simulink model "distributeSystemSim"  (R2017a)
settings: Solver=VariableStepAuto  StartTime=0.0  StopTime=200  RelTol=1e-3
libraries: simulink x3
settings Model: Creator=17423  LastModifiedBy=17423

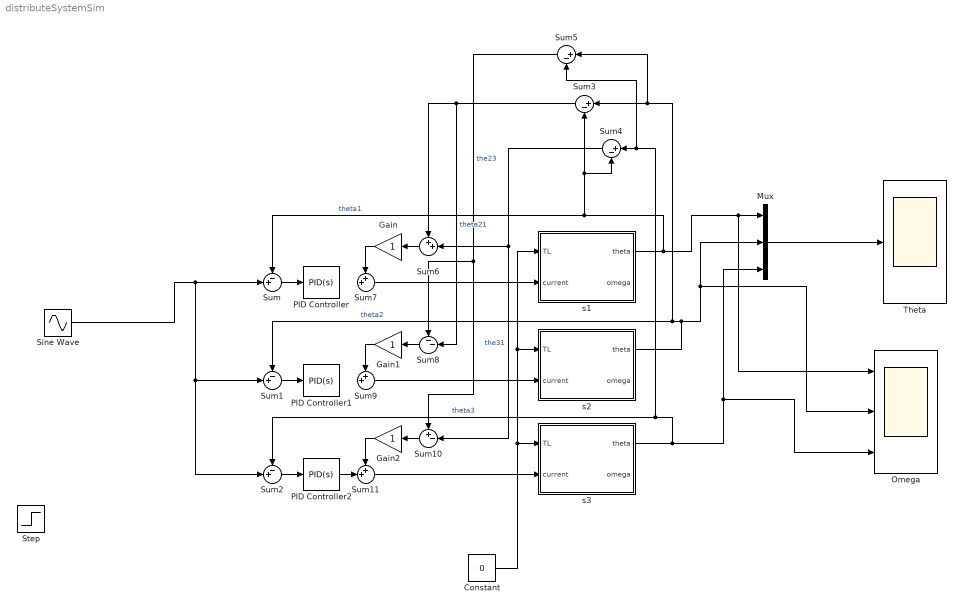
== system distributeSystemSim ==
  Constant : Constant  Value=0
  Gain : Gain
  Gain1 : Gain
  Gain2 : Gain
  Mux : Mux  Inputs=3
  Omega : Scope  NumInputPorts=3
  PID Controller : simulink/Continuous/PID Controller  Controller=PID  TimeDomain=Continuous-time  SampleTime=-1  IntegratorMethod=Forward Euler  FilterMethod=Forward Euler  Form=Parallel  UseFilter=on  ControllerParametersSource=internal  P=0.1  I=0  D=16  N=100  InitialConditionSource=internal  InitialConditionForIntegrator=0  InitialConditionForFilter=0  ExternalReset=none  LimitOutput=off  UpperSaturationLimit=inf  LowerSaturationLimit=-inf  LinearizeAsGain=on  AntiWindupMode=none  Kb=1  TrackingMode=off  Kt=1  PParamMin=[]  PParamMax=[]  IParamMin=[]  IParamMax=[]  DParamMin=[]  DParamMax=[]  NParamMin=[]  NParamMax=[]  KbParamMin=[]  KbParamMax=[]  KtParamMin=[]  KtParamMax=[]  POutMin=[]  POutMax=[]  IOutMin=[]  IOutMax=[]  DOutMin=[]  DOutMax=[]  NOutMin=[]  NOutMax=[]  KbOutMin=[]  KbOutMax=[]  KtOutMin=[]  KtOutMax=[]  IntegratorOutMin=[]  IntegratorOutMax=[]  FilterOutMin=[]  FilterOutMax=[]  SumOutMin=[]  SumOutMax=[]  SumI1OutMin=[]  SumI1OutMax=[]  SumI2OutMin=[]  SumI2OutMax=[]  SumI3OutMin=[]  SumI3OutMax=[]  SumDOutMin=[]  SumDOutMax=[]  SaturationOutMin=[]  SaturationOutMax=[]  IntegratorContinuousStateAttributes=''  IntegratorStateMustResolveToSignalObject=off  IntegratorRTWStateStorageClass=Auto  FilterContinuousStateAttributes=''  FilterStateMustResolveToSignalObject=off  FilterRTWStateStorageClass=Auto  DifferentiatorICPrevScaledInput=0  DifferentiatorOutMin=[]  DifferentiatorOutMax=[]  InitialConditionSetting=State (most efficient)
  PID Controller1 : simulink/Continuous/PID Controller  Controller=PID  TimeDomain=Continuous-time  SampleTime=-1  IntegratorMethod=Forward Euler  FilterMethod=Forward Euler  Form=Parallel  UseFilter=on  ControllerParametersSource=internal  P=0.1  I=0  D=16  N=100  InitialConditionSource=internal  InitialConditionForIntegrator=0  InitialConditionForFilter=0  ExternalReset=none  LimitOutput=off  UpperSaturationLimit=inf  LowerSaturationLimit=-inf  LinearizeAsGain=on  AntiWindupMode=none  Kb=1  TrackingMode=off  Kt=1  PParamMin=[]  PParamMax=[]  IParamMin=[]  IParamMax=[]  DParamMin=[]  DParamMax=[]  NParamMin=[]  NParamMax=[]  KbParamMin=[]  KbParamMax=[]  KtParamMin=[]  KtParamMax=[]  POutMin=[]  POutMax=[]  IOutMin=[]  IOutMax=[]  DOutMin=[]  DOutMax=[]  NOutMin=[]  NOutMax=[]  KbOutMin=[]  KbOutMax=[]  KtOutMin=[]  KtOutMax=[]  IntegratorOutMin=[]  IntegratorOutMax=[]  FilterOutMin=[]  FilterOutMax=[]  SumOutMin=[]  SumOutMax=[]  SumI1OutMin=[]  SumI1OutMax=[]  SumI2OutMin=[]  SumI2OutMax=[]  SumI3OutMin=[]  SumI3OutMax=[]  SumDOutMin=[]  SumDOutMax=[]  SaturationOutMin=[]  SaturationOutMax=[]  IntegratorContinuousStateAttributes=''  IntegratorStateMustResolveToSignalObject=off  IntegratorRTWStateStorageClass=Auto  FilterContinuousStateAttributes=''  FilterStateMustResolveToSignalObject=off  FilterRTWStateStorageClass=Auto  DifferentiatorICPrevScaledInput=0  DifferentiatorOutMin=[]  DifferentiatorOutMax=[]  InitialConditionSetting=State (most efficient)
  PID Controller2 : simulink/Continuous/PID Controller  Controller=PID  TimeDomain=Continuous-time  SampleTime=-1  IntegratorMethod=Forward Euler  FilterMethod=Forward Euler  Form=Parallel  UseFilter=on  ControllerParametersSource=internal  P=0.1  I=0  D=16  N=100  InitialConditionSource=internal  InitialConditionForIntegrator=0  InitialConditionForFilter=0  ExternalReset=none  LimitOutput=off  UpperSaturationLimit=inf  LowerSaturationLimit=-inf  LinearizeAsGain=on  AntiWindupMode=none  Kb=1  TrackingMode=off  Kt=1  PParamMin=[]  PParamMax=[]  IParamMin=[]  IParamMax=[]  DParamMin=[]  DParamMax=[]  NParamMin=[]  NParamMax=[]  KbParamMin=[]  KbParamMax=[]  KtParamMin=[]  KtParamMax=[]  POutMin=[]  POutMax=[]  IOutMin=[]  IOutMax=[]  DOutMin=[]  DOutMax=[]  NOutMin=[]  NOutMax=[]  KbOutMin=[]  KbOutMax=[]  KtOutMin=[]  KtOutMax=[]  IntegratorOutMin=[]  IntegratorOutMax=[]  FilterOutMin=[]  FilterOutMax=[]  SumOutMin=[]  SumOutMax=[]  SumI1OutMin=[]  SumI1OutMax=[]  SumI2OutMin=[]  SumI2OutMax=[]  SumI3OutMin=[]  SumI3OutMax=[]  SumDOutMin=[]  SumDOutMax=[]  SaturationOutMin=[]  SaturationOutMax=[]  IntegratorContinuousStateAttributes=''  IntegratorStateMustResolveToSignalObject=off  IntegratorRTWStateStorageClass=Auto  FilterContinuousStateAttributes=''  FilterStateMustResolveToSignalObject=off  FilterRTWStateStorageClass=Auto  DifferentiatorICPrevScaledInput=0  DifferentiatorOutMin=[]  DifferentiatorOutMax=[]  InitialConditionSetting=State (most efficient)
  Sine Wave : Sin  Amplitude=2  Frequency=0.2  SampleTime=0
  Step : Step  Time=0  SampleTime=0
  Sum : Sum  Inputs=-+|
  Sum1 : Sum  Inputs=-+|
  Sum10 : Sum  Inputs=+-|
  Sum{6..7,9,11} (4 alike) : Sum  Inputs=++|
  Sum2 : Sum  Inputs=-+|
  Sum3 : Sum  Inputs=|+-
  Sum4 : Sum  Inputs=|+-
  Sum5 : Sum  Inputs=|+-
  Sum8 : Sum  Inputs=--|
  Theta : Scope
  s1 : Subsystem
  s2 : Subsystem
  s3 : Subsystem
  wires:
  Constant/1 -> s1/1(TL), s2/1(TL), s3/1(TL)
  Mux/1 -> Theta/1
  Sum/1 -> PID Controller/1
  s1/1(theta) -> Omega/1, Mux/1, Sum/1, Sum4/2, Sum3/2  "theta1"
  Sine Wave/1 -> Sum2/2, Sum1/2, Sum/2
  s2/1(theta) -> Omega/2, Mux/2, Sum5/1, Sum3/1, Sum1/1  "theta2"
  Sum1/1 -> PID Controller1/1
  s3/1(theta) -> Omega/3, Mux/3, Sum5/2, Sum4/1, Sum2/1  "theta3"
  Sum2/1 -> PID Controller2/1
  Sum3/1 -> Sum8/2, Sum6/1  "theta21"
  Sum4/1 -> Sum10/2, Sum6/2  "the31"
  Sum6/1 -> Gain/1
  Gain/1 -> Sum7/1
  Sum7/1 -> s1/2(current)
  PID Controller2/1 -> Sum11/2
  Gain2/1 -> Sum11/1
  Gain1/1 -> Sum9/1
  Sum5/1 -> Sum10/1, Sum8/1  "the23"
  Sum8/1 -> Gain1/1
  Sum9/1 -> s2/2(current)
  Sum10/1 -> Gain2/1
  Sum11/1 -> s3/2(current)

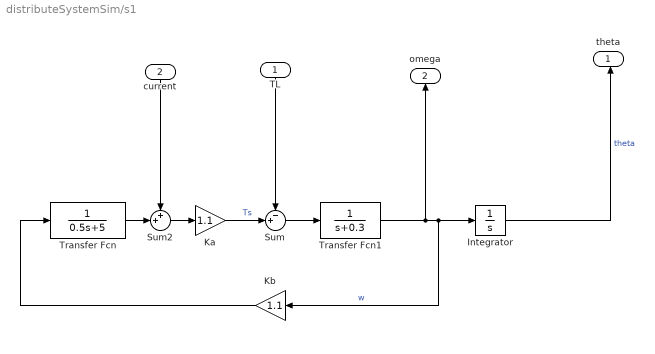
== system distributeSystemSim/s1 ==
  TL : Inport
  current : Inport  Port=2
  Integrator : Integrator  InitialCondition=-1
  Ka : Gain  Gain=1.1
  Kb : Gain  Gain=1.1
  Sum : Sum  Inputs=-+|
  Sum2 : Sum  Inputs=++|
  Transfer Fcn : TransferFcn  Denominator=[0.5 5]
  Transfer Fcn1 : TransferFcn  Denominator=[1 0.3]
  theta : Outport
  omega : Outport  Port=2
  wires:
  current/1 -> Sum2/1
  Sum2/1 -> Ka/1
  Ka/1 -> Sum/2  "Ts"
  Sum/1 -> Transfer Fcn1/1
  TL/1 -> Sum/1
  Transfer Fcn1/1 -> omega/1, Kb/1, Integrator/1  "w"
  Transfer Fcn/1 -> Sum2/2
  Kb/1 -> Transfer Fcn/1
  Integrator/1 -> theta/1  "theta"

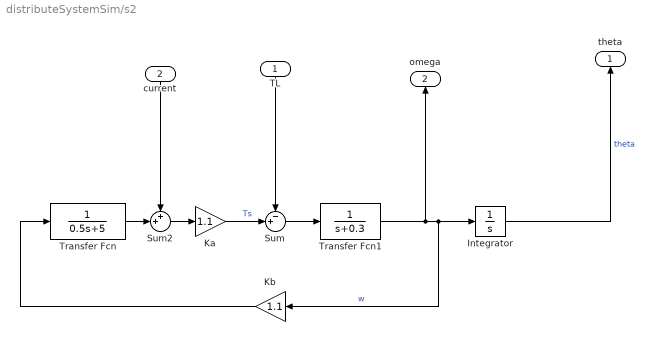
== system distributeSystemSim/s2 ==
  TL : Inport
  current : Inport  Port=2
  Integrator : Integrator  InitialCondition=-2
  Ka : Gain  Gain=1.1
  Kb : Gain  Gain=1.1
  Sum : Sum  Inputs=-+|
  Sum2 : Sum  Inputs=++|
  Transfer Fcn : TransferFcn  Denominator=[0.5 5]
  Transfer Fcn1 : TransferFcn  Denominator=[1 0.3]
  theta : Outport
  omega : Outport  Port=2
  wires:
  Integrator/1 -> theta/1  "theta"
  Kb/1 -> Transfer Fcn/1
  Transfer Fcn/1 -> Sum2/2
  Transfer Fcn1/1 -> Integrator/1, Kb/1, omega/1  "w"
  TL/1 -> Sum/1
  Sum/1 -> Transfer Fcn1/1
  Ka/1 -> Sum/2  "Ts"
  Sum2/1 -> Ka/1
  current/1 -> Sum2/1

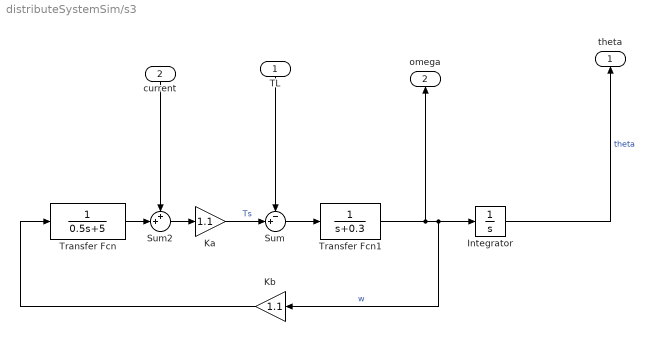
== system distributeSystemSim/s3 ==
  TL : Inport
  current : Inport  Port=2
  Integrator : Integrator
  Ka : Gain  Gain=1.1
  Kb : Gain  Gain=1.1
  Sum : Sum  Inputs=-+|
  Sum2 : Sum  Inputs=++|
  Transfer Fcn : TransferFcn  Denominator=[0.5 5]
  Transfer Fcn1 : TransferFcn  Denominator=[1 0.3]
  theta : Outport
  omega : Outport  Port=2
  wires:
  current/1 -> Sum2/1
  Sum2/1 -> Ka/1
  Ka/1 -> Sum/2  "Ts"
  Sum/1 -> Transfer Fcn1/1
  TL/1 -> Sum/1
  Transfer Fcn1/1 -> omega/1, Kb/1, Integrator/1  "w"
  Transfer Fcn/1 -> Sum2/2
  Kb/1 -> Transfer Fcn/1
  Integrator/1 -> theta/1  "theta"
